simulink model "BEV_maxSpeed"  (R2023a)
settings: Solver=FixedStepAuto  StartTime=0.0  StopTime=1000  FixedStep=1  RelTol=1e-3
undefined symbols (not defined in the file): acceleration_threshold, attributes, battery_GD, config_gearbox, config_Inverter, config_motor, config_vehicle, efficiency_vector, efficiency_vector2, GB, gearbox_map, k_FW, lossData, lossData2, max_torque_map, max_torque_map2, speed_vector, speed_vector2
libraries: spsParallelRLCBranchLib x20, spsControlledCurrentSourceLib x8, spsVoltageMeasurementLib x8, simulink x4, spsDCVoltageSourceLib x4, spspowerguiLib x4, eePmsmCurrentReferenceGen x2
(part 2 of 2)

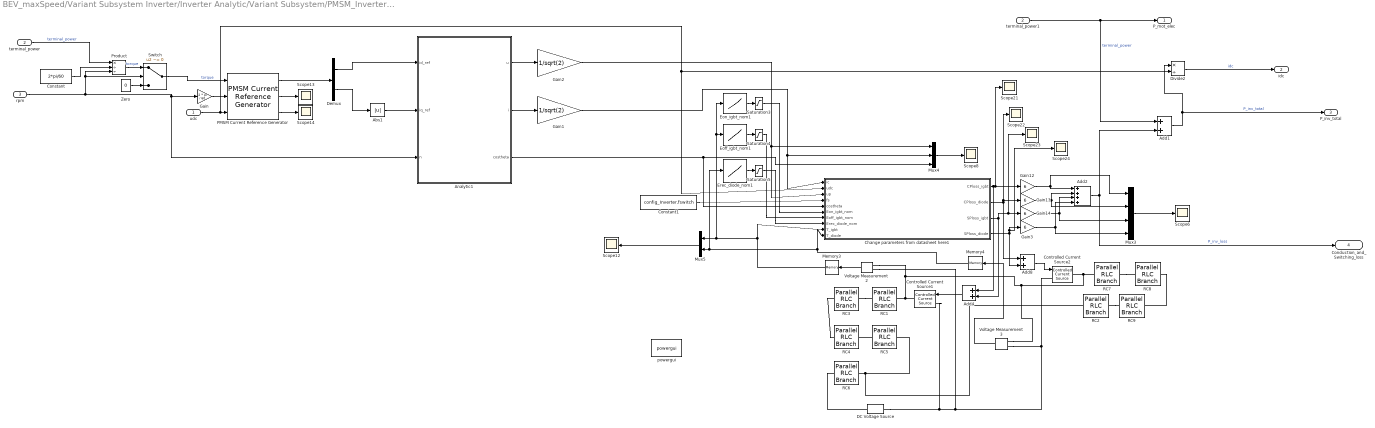
== system BEV_maxSpeed/Variant Subsystem Inverter/Inverter Analytic/Variant Subsystem/PMSM_Inverter_IBGT_Analytic ==
  udc : Inport
  terminal_power : Inport  Port=2
  rpm : Inport  Port=3
  Abs1 : Abs  SaturateOnIntegerOverflow=off
  Add1 : Sum
  Add2 : Sum  Inputs=++++
  Add4 : Sum
  Add8 : Sum
  Analytic1 : MATLAB Function  TreatAsAtomicUnit=on
  Change parameters from datasheet here1 : MATLAB Function  TreatAsAtomicUnit=on
  Constant : Constant  Value=2*pi/60
  Constant1 : Constant  Value=config_Inverter.fswitch
  Controlled Current Source1 : spsControlledCurrentSourceLib/Controlled Current Source  Initialize=on  Source_Type=AC  Amplitude=0  Phase=0  Frequency=0  Measurements=None
  Controlled Current Source2 : spsControlledCurrentSourceLib/Controlled Current Source  Initialize=on  Source_Type=AC  Amplitude=0  Phase=0  Frequency=0  Measurements=None
  DC Voltage Source : spsDCVoltageSourceLib/DC Voltage Source  Amplitude=25  Measurements=None
  Demux : Demux  Outputs=2
  Divide2 : Product  Inputs=*/
  Eoff_igbt_nom1 : Lookup_n-D  NumberOfTableDimensions=1  BreakpointsForDimension1=[25, 150, 175]  Table="[23.5*1e-3,  29*1e-3,  30*1e-3]"  InternalRulePriority=Speed  RndMeth=Simplest
  Eon_igbt_nom1 : Lookup_n-D  NumberOfTableDimensions=1  BreakpointsForDimension1=[25, 150, 175]  Table="[13.5*1e-3,  17.5*1e-3,  18*1e-3]"  InternalRulePriority=Speed  RndMeth=Simplest
  Erec_diode_nom1 : Lookup_n-D  NumberOfTableDimensions=1  BreakpointsForDimension1=[25, 150, 175]  Table="[7*1e-3,  13*1e-3,  15*1e-3]"  InternalRulePriority=Speed  RndMeth=Simplest
  Gain : Gain  Gain=2 * pi / 60
  Gain1 : Gain  Gain=1/sqrt(2)
  Gain{3,12..14} (4 alike) : Gain  Gain=6
  Gain2 : Gain  Gain=1/sqrt(2)
  Memory3 : Memory  InitialCondition=25  InheritSampleTime=on
  Memory4 : Memory  InitialCondition=25  InheritSampleTime=on
  Mux3 : Mux
  Mux4 : Mux  Inputs=3
  Mux5 : Mux  Inputs=2
  PMSM Current Reference Generator : eePmsmCurrentReferenceGen/PMSM Current Reference Generator  Vnom=360  Pmax=150000  Tmax=350  Ts=-1  RefType=Automatically generated lookup-table  rpmVec=[0, 3000]  TqVec=[-100, 0, 100]  VdcVec=[300, 350]  PWMMode=SPWM: sinusoidal PWM  ModFactor=0.97  idMatrix=zeros(2,3,2)  iqMatrix=zeros(2,3,2)  p=6  psim=0.0347  Ld=0.0000436  Lq=0.0000975  Rs=0.0049  RefExpEnable=0
      settings: LibrarySourceBlock=|
      | ee_sl_lib/PMSM Control/PMSM Current Reference
      | Generator
  Product : Product  Inputs=*//
  RC1 : spsParallelRLCBranchLib/Parallel RLC Branch  LConnTagsString=a  RConnTagsString=__new0  BranchType=RC  Resistance=config_Inverter.R1igbt  Inductance=1e-3  SetiL0=off  InitialCurrent=0  Capacitance=config_Inverter.C1igbt  Setx0=off  InitialVoltage=0  Measurements=None
  RC2 : spsParallelRLCBranchLib/Parallel RLC Branch  LConnTagsString=a  RConnTagsString=__new0  BranchType=RC  Resistance=config_Inverter.R4diode  Inductance=1e-3  SetiL0=off  InitialCurrent=0  Capacitance=config_Inverter.C4diode  Setx0=off  InitialVoltage=0  Measurements=None
  RC3 : spsParallelRLCBranchLib/Parallel RLC Branch  LConnTagsString=a  RConnTagsString=__new0  BranchType=RC  Resistance=config_Inverter.R2igbt  Inductance=1e-3  SetiL0=off  InitialCurrent=0  Capacitance=config_Inverter.C2igbt  Setx0=off  InitialVoltage=0  Measurements=None
  RC4 : spsParallelRLCBranchLib/Parallel RLC Branch  LConnTagsString=a  RConnTagsString=__new0  BranchType=RC  Resistance=config_Inverter.R3igbt  Inductance=1e-3  SetiL0=off  InitialCurrent=0  Capacitance=config_Inverter.C3igbt  Setx0=off  InitialVoltage=0  Measurements=None
  RC5 : spsParallelRLCBranchLib/Parallel RLC Branch  LConnTagsString=a  RConnTagsString=__new0  BranchType=RC  Resistance=config_Inverter.R4igbt  Inductance=1e-3  SetiL0=off  InitialCurrent=0  Capacitance=config_Inverter.C4igbt  Setx0=off  InitialVoltage=0  Measurements=None
  RC6 : spsParallelRLCBranchLib/Parallel RLC Branch  LConnTagsString=a  RConnTagsString=__new0  BranchType=R  Resistance=config_Inverter.R6igbt  Inductance=1e-3  SetiL0=off  InitialCurrent=0  Capacitance=175  Setx0=on  InitialVoltage=0  Measurements=None
  RC7 : spsParallelRLCBranchLib/Parallel RLC Branch  LConnTagsString=a  RConnTagsString=__new0  BranchType=RC  Resistance=config_Inverter.R1diode  Inductance=1e-3  SetiL0=off  InitialCurrent=0  Capacitance=config_Inverter.C1diode  Setx0=off  InitialVoltage=0  Measurements=None
  RC8 : spsParallelRLCBranchLib/Parallel RLC Branch  LConnTagsString=a  RConnTagsString=__new0  BranchType=RC  Resistance=config_Inverter.R2diode  Inductance=1e-3  SetiL0=off  InitialCurrent=0  Capacitance=config_Inverter.C2diode  Setx0=off  InitialVoltage=0  Measurements=None
  RC9 : spsParallelRLCBranchLib/Parallel RLC Branch  LConnTagsString=a  RConnTagsString=__new0  BranchType=RC  Resistance=config_Inverter.R3diode  Inductance=1e-3  SetiL0=off  InitialCurrent=0  Capacitance=config_Inverter.C3diode  Setx0=off  InitialVoltage=0  Measurements=None
  Saturation3 : Saturate  UpperLimit=18*1e-3  LowerLimit=13.5*1e-3
  Saturation4 : Saturate  UpperLimit=30*1e-3  LowerLimit=23.5*1e-3
  Saturation5 : Saturate  UpperLimit=15*1e-3  LowerLimit=7*1e-3
  Scope{6,8,12..14,21..24} (9 alike) : Scope
  Switch : Switch  Criteria=u2 ~= 0  SaturateOnIntegerOverflow=off  InputSameDT=off
  Voltage Measurement2 : spsVoltageMeasurementLib/Voltage Measurement  PhasorSimulation=off  OutputType=Complex  PSBequivalent=0
  Voltage Measurement3 : spsVoltageMeasurementLib/Voltage Measurement  PhasorSimulation=off  OutputType=Complex  PSBequivalent=0
  Zero : Constant  Value=0  OutDataTypeStr=Inherit: Inherit via back propagation
  powergui : spspowerguiLib/powergui  Priority=1  SimulationMode=Discrete  SampleTime=1  frequency=60  Iterations=50  frequencyindice=0  Pbase=100e6  ErrMax=1e-4  UnitsV=kV  UnitsW=MW  buscounter=0  FunctionMessages=on  echomessages=on  EnableUseOfTLC=off  CurrentSourceSwitches=off  DisableSnubberDevices=off  DisableRonSwitches=off  DisableVfSwitches=off  DisplayEquations=off  AutomaticDiscreteSolvers=off  SolverType=Backward Euler  Interpol=off  ExternalGateDelay=off  methode=off  Ts=100  x0status=blocks  SPID=off  SwTol=0  HookPort=off  NonlinearTolerance=1e-4  nMaxIteration=100  ContinueOnMaxIteration=off  RestoreLinks=warning  ResistiveCurrentMeasurement=off  Frange=[0:2:500]  Ylog=off  Xlog=on  ShowGrid=off  save=off  variable=ZData  structure=0  ZoomFFT=off  StartTime=0.0  cycles=1  DisplayStyle=1  fundamental=60  FreqAxis=off  MaxFrequency=1000  frequencyindicesteady=1  RmsSteady=1  display=off
  terminal_power1 : InportShadow  Port=2
  P_mot_elec : Outport
  idc : Outport  Port=2
  P_inv_total : Outport  Port=3
  Conduction_and_Switching_loss : Outport  Port=4
  wires:
  PMSM Current Reference Generator/2 -> Scope13/1
  Eon_igbt_nom1/1 -> Saturation3/1
  Divide2/1 -> idc/1  "idc"
  Voltage Measurement2/1 -> Memory3/1
  Add8/1 -> Controlled Current Source2/1
  Change parameters from datasheet here1/3(SPloss_igbt) -> Scope23/1, Gain14/1, Add4/2
  Change parameters from datasheet here1/1(CPloss_igbt) -> Add4/1, Gain12/1, Scope21/1
  Gain2/1 -> Change parameters from datasheet here1/3(up), Mux4/1
  Add4/1 -> Controlled Current Source1/1
  Constant1/1 -> Change parameters from datasheet here1/4(fs)
  Eoff_igbt_nom1/1 -> Saturation4/1
  Saturation4/1 -> Change parameters from datasheet here1/7(Eoff_igbt_nom)
  PMSM Current Reference Generator/3 -> Scope14/1
  Demux/2 -> Abs1/1
  Change parameters from datasheet here1/2(CPloss_diode) -> Scope22/1, Gain13/1, Add8/1
  Voltage Measurement3/1 -> Memory4/1
  Memory3/1 -> Change parameters from datasheet here1/9(T_igbt), Eoff_igbt_nom1/1, Eon_igbt_nom1/1, Mux5/1
  Mux4/1 -> Scope8/1
  Mux5/1 -> Scope12/1
  Demux/1 -> Analytic1/1(id_ref)
  Memory4/1 -> Erec_diode_nom1/1, Mux5/2, Change parameters from datasheet here1/10(T_diode)
  Saturation5/1 -> Change parameters from datasheet here1/8(Erec_diode_nom)
  Add1/1 -> Divide2/1, P_inv_total/1  "P_inv_total"
  Analytic1/1(u) -> Gain2/1
  Erec_diode_nom1/1 -> Saturation5/1
  Mux3/1 -> Scope6/1
  Gain14/1 -> Mux3/3, Add2/3
  Gain/1 -> PMSM Current Reference Generator/2
  Add2/1 -> Conduction_and_Switching_loss/1, Add1/2  "P_inv_loss"
  Change parameters from datasheet here1/4(SPloss_diode) -> Scope24/1, Gain3/1, Add8/2
  Analytic1/2(i) -> Gain1/1
  PMSM Current Reference Generator/1 -> Demux/1
  Saturation3/1 -> Change parameters from datasheet here1/6(Eon_igbt_nom)
  Abs1/1 -> Analytic1/2(iq_ref)
  Gain13/1 -> Mux3/2, Add2/2
  rpm/1 -> Switch/2, Product/3, Analytic1/3(n), Gain/1
  terminal_power1/1 -> P_mot_elec/1, Add1/1  "terminal_power"
  Gain1/1 -> Change parameters from datasheet here1/1(ic), Mux4/2
  Gain12/1 -> Mux3/1, Add2/1
  udc/1 -> PMSM Current Reference Generator/3, Change parameters from datasheet here1/2(udc), Divide2/2
  Switch/1 -> PMSM Current Reference Generator/1  "torque"
  Gain3/1 -> Add2/4, Mux3/4
  Analytic1/3(costheta) -> Mux4/3, Change parameters from datasheet here1/5(costheta)
  terminal_power/1 -> Product/1  "terminal_power"
  Constant/1 -> Product/2
  Product/1 -> Switch/1  "torque"
  Zero/1 -> Switch/3
  connections:
  RC3/RConn1 -- RC1/LConn1
  RC7/LConn1 -- RC8/RConn1
  DC Voltage Source/RConn1 -- RC6/LConn1
  RC3/LConn1 -- RC4/LConn1
  RC5/LConn1 -- RC4/RConn1
  RC8/LConn1 -- RC9/LConn1
  Controlled Current Source1/LConn1 -- DC Voltage Source/LConn1 -- Voltage Measurement2/LConn1 -- Voltage Measurement3/LConn1 -- Controlled Current Source2/LConn1
  RC2/LConn1 -- RC9/RConn1
  RC5/RConn1 -- RC6/RConn1 -- RC2/RConn1
  Controlled Current Source2/RConn1 -- RC7/RConn1 -- Voltage Measurement3/LConn2 -- Voltage Measurement2/LConn2 -- Controlled Current Source1/RConn1 -- RC1/RConn1

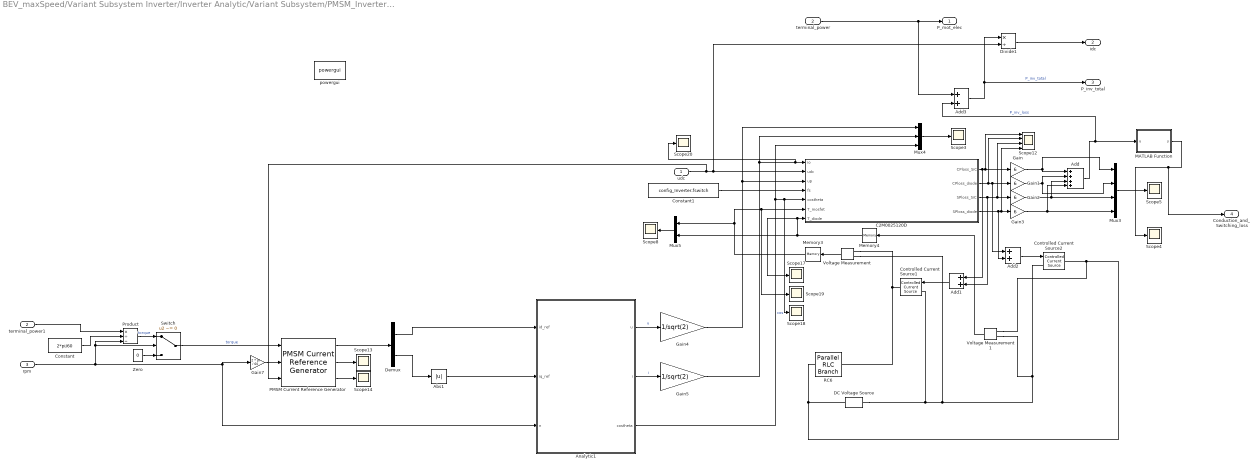
== system BEV_maxSpeed/Variant Subsystem Inverter/Inverter Analytic/Variant Subsystem/PMSM_Inverter_SiC-MOSFET_Analytic ==
  udc : Inport
  terminal_power : Inport  Port=2
  rpm : Inport  Port=3
  Abs1 : Abs  SaturateOnIntegerOverflow=off
  Add : Sum  Inputs=++++
  Add1 : Sum
  Add2 : Sum
  Add3 : Sum
  Analytic1 : MATLAB Function  TreatAsAtomicUnit=on
  C2M0025120D : MATLAB Function  TreatAsAtomicUnit=on
  Constant : Constant  Value=2*pi/60
  Constant1 : Constant  Value=config_Inverter.fswitch
  Controlled Current Source1 : spsControlledCurrentSourceLib/Controlled Current Source  Initialize=on  Source_Type=AC  Amplitude=0  Phase=0  Frequency=0  Measurements=None
  Controlled Current Source2 : spsControlledCurrentSourceLib/Controlled Current Source  Initialize=on  Source_Type=AC  Amplitude=0  Phase=0  Frequency=0  Measurements=None
  DC Voltage Source : spsDCVoltageSourceLib/DC Voltage Source  Amplitude=25  Measurements=None
  Demux : Demux  Outputs=2
  Divide1 : Product  Inputs=*/
  Gain{,1..3} (4 alike) : Gain  Gain=6
  Gain4 : Gain  Gain=1/sqrt(2)
  Gain5 : Gain  Gain=1/sqrt(2)
  Gain7 : Gain  Gain=2 * pi / 60
  MATLAB Function : MATLAB Function  TreatAsAtomicUnit=on
  Memory3 : Memory  InitialCondition=25  InheritSampleTime=on
  Memory4 : Memory  InitialCondition=25  InheritSampleTime=on
  Mux3 : Mux
  Mux4 : Mux  Inputs=3
  Mux5 : Mux  Inputs=2
  PMSM Current Reference Generator : eePmsmCurrentReferenceGen/PMSM Current Reference Generator  Vnom=360  Pmax=150000  Tmax=350  Ts=-1  RefType=Automatically generated lookup-table  rpmVec=[0, 3000]  TqVec=[-100, 0, 100]  VdcVec=[300, 350]  PWMMode=SPWM: sinusoidal PWM  ModFactor=0.97  idMatrix=zeros(2,3,2)  iqMatrix=zeros(2,3,2)  p=6  psim=0.0347  Ld=0.0000436  Lq=0.0000975  Rs=0.0049  RefExpEnable=0
      settings: LibrarySourceBlock=|
      | ee_sl_lib/PMSM Control/PMSM Current Reference
      | Generator
  Product : Product  Inputs=*//
  RC6 : spsParallelRLCBranchLib/Parallel RLC Branch  LConnTagsString=a  RConnTagsString=__new0  BranchType=R  Resistance=config_Inverter.Rmosfet  Inductance=1e-3  SetiL0=off  InitialCurrent=0  Capacitance=175  Setx0=on  InitialVoltage=0  Measurements=None
  Scope12 : Scope  NumInputPorts=4
  Scope{3..5,8,13..14,17..20} (10 alike) : Scope
  Switch : Switch  Criteria=u2 ~= 0  SaturateOnIntegerOverflow=off  InputSameDT=off
  Voltage Measurement : spsVoltageMeasurementLib/Voltage Measurement  PhasorSimulation=off  OutputType=Complex  PSBequivalent=0
  Voltage Measurement1 : spsVoltageMeasurementLib/Voltage Measurement  PhasorSimulation=off  OutputType=Complex  PSBequivalent=0
  Zero : Constant  Value=0  OutDataTypeStr=Inherit: Inherit via back propagation
  powergui : spspowerguiLib/powergui  Priority=1  SimulationMode=Discrete  SampleTime=1  frequency=60  Iterations=50  frequencyindice=0  Pbase=100e6  ErrMax=1e-4  UnitsV=kV  UnitsW=MW  buscounter=0  FunctionMessages=on  echomessages=on  EnableUseOfTLC=off  CurrentSourceSwitches=off  DisableSnubberDevices=off  DisableRonSwitches=off  DisableVfSwitches=off  DisplayEquations=off  AutomaticDiscreteSolvers=off  SolverType=Backward Euler  Interpol=off  ExternalGateDelay=off  methode=off  Ts=100  x0status=blocks  SPID=off  SwTol=0  HookPort=off  NonlinearTolerance=1e-4  nMaxIteration=100  ContinueOnMaxIteration=off  RestoreLinks=warning  ResistiveCurrentMeasurement=off  Frange=[0:2:500]  Ylog=off  Xlog=on  ShowGrid=off  save=off  variable=ZData  structure=0  ZoomFFT=off  StartTime=0.0  cycles=1  DisplayStyle=1  fundamental=60  FreqAxis=off  MaxFrequency=1000  frequencyindicesteady=1  RmsSteady=1  display=off
  terminal_power1 : InportShadow  Port=2
  P_mot_elec : Outport
  idc : Outport  Port=2
  P_inv_total : Outport  Port=3
  Conduction_and_Switching_loss : Outport  Port=4
  wires:
  udc/1 -> PMSM Current Reference Generator/3, Divide1/2, C2M0025120D/2(udc)
  Gain1/1 -> Mux3/2, Add/2
  Gain4/1 -> Mux4/1, C2M0025120D/3(up)
  Memory3/1 -> Mux5/1, Scope19/1, C2M0025120D/6(T_mosfet)
  Add2/1 -> Controlled Current Source2/1
  Constant1/1 -> C2M0025120D/4(fs)
  Divide1/1 -> idc/1
  C2M0025120D/3(SPloss_SiC) -> Add1/2, Scope12/3, Gain2/1
  Analytic1/3(costheta) -> Mux4/3, Scope18/1, C2M0025120D/5(costheta)  "cos"
  Gain/1 -> Mux3/1, Add/1
  C2M0025120D/2(CPloss_diode) -> Scope12/2, Add2/1, Gain1/1
  Mux4/1 -> Scope3/1
  Gain5/1 -> Mux4/2, Scope20/1, C2M0025120D/1(io)
  terminal_power/1 -> P_mot_elec/1, Add3/1
  Memory4/1 -> Scope17/1, C2M0025120D/7(T_diode), Mux5/2
  Add/1 -> Add3/2, MATLAB Function/1(u)  "P_inv_loss"
  C2M0025120D/4(SPloss_diode) -> Scope12/4, Gain3/1, Add2/2
  Gain2/1 -> Mux3/3, Add/3
  Add1/1 -> Controlled Current Source1/1
  C2M0025120D/1(CPloss_SiC) -> Add1/1, Scope12/1, Gain/1
  Analytic1/2(i) -> Gain5/1  "i"
  Gain3/1 -> Add/4, Mux3/4
  Voltage Measurement1/1 -> Memory4/1
  Add3/1 -> P_inv_total/1, Divide1/1  "P_inv_total"
  Voltage Measurement/1 -> Memory3/1
  Mux5/1 -> Scope8/1
  Mux3/1 -> Scope5/1
  Analytic1/1(u) -> Gain4/1  "u"
  PMSM Current Reference Generator/3 -> Scope14/1
  PMSM Current Reference Generator/2 -> Scope13/1
  Switch/1 -> PMSM Current Reference Generator/1  "torque"
  Demux/2 -> Abs1/1
  rpm/1 -> Gain7/1, Analytic1/3(n), Switch/2, Product/3
  Gain7/1 -> PMSM Current Reference Generator/2
  Demux/1 -> Analytic1/1(id_ref)
  Abs1/1 -> Analytic1/2(iq_ref)
  PMSM Current Reference Generator/1 -> Demux/1
  Zero/1 -> Switch/3
  Constant/1 -> Product/2
  Product/1 -> Switch/1  "torque"
  terminal_power1/1 -> Product/1
  MATLAB Function/1(y) -> Conduction_and_Switching_loss/1, Scope4/1
  connections:
  Voltage Measurement/LConn1 -- Controlled Current Source1/RConn1 -- RC6/RConn1
  DC Voltage Source/RConn1 -- Controlled Current Source2/RConn1 -- Voltage Measurement1/LConn1 -- RC6/LConn1
  Voltage Measurement1/LConn2 -- DC Voltage Source/LConn1 -- Controlled Current Source1/LConn1 -- Voltage Measurement/LConn2 -- Controlled Current Source2/LConn1

== system BEV_maxSpeed/Variant Subsystem Gearbox/Gearbox Analytic/Variant Subsystem Analytic GB/Einstufig_Achsparallel/Ölpumpe ==
  nrad : Inport
  Constant : Constant  Value=config_gearbox.power_oilpump
  Constant1 : Constant  Value=1.5e3
  Product : Product  Inputs=*/*
  Scope : Scope
  power_oilpump : Outport
  wires:
  Product/1 -> power_oilpump/1, Scope/1
  Constant1/1 -> Product/2
  nrad/1 -> Product/1
  Constant/1 -> Product/3

== system BEV_maxSpeed/Variant Subsystem Gearbox/Gearbox Analytic/Variant Subsystem Analytic GB/Zweistufig_Achsparallel/Ölpumpe ==
  nrad : Inport
  Constant : Constant  Value=config_gearbox.power_oilpump
  Constant1 : Constant  Value=15e3
  Product : Product  Inputs=*/*
  Scope : Scope
  power_oilpump : Outport
  wires:
  Product/1 -> power_oilpump/1, Scope/1
  Constant1/1 -> Product/2
  nrad/1 -> Product/1
  Constant/1 -> Product/3

== system BEV_maxSpeed/Variant Subsystem Gearbox/Gearbox Analytic/Variant Subsystem Analytic GB/Zweistufig_Koaxial/Ölpumpe ==
  nrad : Inport
  Constant : Constant  Value=config_gearbox.power_oilpump
  Constant1 : Constant  Value=1.5e3
  Product : Product  Inputs=*/*
  Scope : Scope
  power_oilpump : Outport
  wires:
  Product/1 -> power_oilpump/1, Scope/1
  Constant1/1 -> Product/2
  nrad/1 -> Product/1
  Constant/1 -> Product/3

== system BEV_maxSpeed/Variant Subsystem Gearbox/Gearbox Lookup-Table/Variant Subsystem/ETA_map/Lookup Gearbox ==
  note: 1) Add Subsystem or Model blocks as valid variant choices.
      | 2) You cannot connect blocks at this level. At simulation, connectivity is automatically
      | determined, based on the active variant and port name matching.
  Torque : Inport
  RPM : Inport  Port=2
  Temp : Inport  Port=3
  Lookup with Temp : Subsystem  VariantControl=gearbox_map.dim_lookup == 3
  Lookup without Temp : Subsystem  VariantControl=gearbox_map.dim_lookup == 2
  Eta : Outport

== system BEV_maxSpeed/Variant Subsystem Gearbox/Gearbox Lookup-Table/Variant Subsystem/ETA_map/Oilpump ==
  rpm_wheel : Inport
  Constant7 : Constant  Value=config_gearbox.power_oilpump
  Constant8 : Constant  Value=1.5e3
  Product4 : Product  Inputs=**/
  loss_oilpump : Outport
  wires:
  rpm_wheel/1 -> Product4/1
  Constant8/1 -> Product4/3
  Constant7/1 -> Product4/2
  Product4/1 -> loss_oilpump/1  "loss_oilpump"

== system BEV_maxSpeed/Variant Subsystem Gearbox/Gearbox Lookup-Table/Variant Subsystem/LOSS_map/Lookup Gearbox ==
  note: 1) Add Subsystem or Model blocks as valid variant choices.
      | 2) You cannot connect blocks at this level. At simulation, connectivity is automatically
      | determined, based on the active variant and port name matching.
  Torque : Inport
  RPM : Inport  Port=2
  Temp : Inport  Port=3
  Lookup with Temp : Subsystem  VariantControl=gearbox_map.dim_lookup == 3
  Lookup without Temp : Subsystem  VariantControl=gearbox_map.dim_lookup == 2
  Loss : Outport

== system BEV_maxSpeed/Variant Subsystem Gearbox/Gearbox Lookup-Table/Variant Subsystem/LOSS_map/Oilpump ==
  rpm_wheel : Inport
  Constant7 : Constant  Value=config_gearbox.power_oilpump
  Constant8 : Constant  Value=1.5e3
  Product4 : Product  Inputs=**/
  loss_oilpump : Outport
  wires:
  Product4/1 -> loss_oilpump/1  "loss_oilpump"
  Constant7/1 -> Product4/2
  Constant8/1 -> Product4/3
  rpm_wheel/1 -> Product4/1

== system BEV_maxSpeed/Variant Subsystem Gearbox/Gearbox Lookup-Table/Variant Subsystem/ETA_map/Lookup Gearbox/Lookup with Temp ==
  Torque : Inport
  RPM : Inport  Port=2
  Temp : Inport  Port=3
  n-D Lookup Table : Lookup_n-D  NumberOfTableDimensions=3  BreakpointsForDimension1=gearbox_map.torque  BreakpointsForDimension2=gearbox_map.rpm  BreakpointsForDimension3=gearbox_map.temperature  Table=gearbox_map.eta  UseLastTableValue=on  InternalRulePriority=Speed  RndMeth=Simplest
      settings: InputPortMap=u0,u1,u2
  Eta : Outport
  wires:
  Torque/1 -> n-D Lookup Table/1
  RPM/1 -> n-D Lookup Table/2
  Temp/1 -> n-D Lookup Table/3
  n-D Lookup Table/1 -> Eta/1

== system BEV_maxSpeed/Variant Subsystem Gearbox/Gearbox Lookup-Table/Variant Subsystem/ETA_map/Lookup Gearbox/Lookup without Temp ==
  Torque : Inport
  RPM : Inport  Port=2
  n-D Lookup Table : Lookup_n-D  BreakpointsForDimension1=gearbox_map.torque  BreakpointsForDimension2=gearbox_map.rpm  BreakpointsForDimension3=gearbox_map.temperature  Table=gearbox_map.eta  UseLastTableValue=on  InternalRulePriority=Speed  RndMeth=Simplest
      settings: InputPortMap=u0,u1
  Eta : Outport
  wires:
  Torque/1 -> n-D Lookup Table/1
  RPM/1 -> n-D Lookup Table/2
  n-D Lookup Table/1 -> Eta/1

== system BEV_maxSpeed/Variant Subsystem Gearbox/Gearbox Lookup-Table/Variant Subsystem/LOSS_map/Lookup Gearbox/Lookup with Temp ==
  Torque : Inport
  RPM : Inport  Port=2
  Temp : Inport  Port=3
  n-D Lookup Table : Lookup_n-D  NumberOfTableDimensions=3  BreakpointsForDimension1=gearbox_map.torque  BreakpointsForDimension2=gearbox_map.rpm  BreakpointsForDimension3=gearbox_map.temperature  Table=gearbox_map.loss  UseLastTableValue=on  InternalRulePriority=Speed  RndMeth=Simplest
      settings: InputPortMap=u0,u1,u2
  Loss : Outport
  wires:
  n-D Lookup Table/1 -> Loss/1
  Temp/1 -> n-D Lookup Table/3
  RPM/1 -> n-D Lookup Table/2
  Torque/1 -> n-D Lookup Table/1

== system BEV_maxSpeed/Variant Subsystem Gearbox/Gearbox Lookup-Table/Variant Subsystem/LOSS_map/Lookup Gearbox/Lookup without Temp ==
  Torque : Inport
  RPM : Inport  Port=2
  n-D Lookup Table : Lookup_n-D  BreakpointsForDimension1=gearbox_map.torque  BreakpointsForDimension2=gearbox_map.rpm  BreakpointsForDimension3=gearbox_map.temperature  Table=gearbox_map.loss  UseLastTableValue=on  InternalRulePriority=Speed  RndMeth=Simplest
      settings: InputPortMap=u0,u1
  Loss : Outport
  wires:
  n-D Lookup Table/1 -> Loss/1
  RPM/1 -> n-D Lookup Table/2
  Torque/1 -> n-D Lookup Table/1

== matlab function BEV_maxSpeed/MATLAB Function ==
  data: availble_torque_acc_motor input; a output; iges input; tire_radius input; mass_total input
function a = fcn(availble_torque_acc_motor, iges, tire_radius, mass_total)

 torque_wheel = availble_torque_acc_motor * iges;

 F_net = torque_wheel / tire_radius;

 a = F_net / mass_total;

== matlab function BEV_maxSpeed/MATLAB Function1 ==
  data: a input; dt input; v_new output; v_prev input; time_prev input; time_new output
function [v_new, time_new] = update_velocity(a, dt, v_prev, time_prev)
    % Inputs:
    % a          - Acceleration (input signal)
    % dt         - Time step (constant or input signal)
    % v_prev     - Previous velocity (feedback input)
    % time_prev  - Previous time (feedback input)

    % Outputs:
    % v_new     - Updated velocity
    % time_new  - Updated time

    % Calculate new velocity using v = u + a * dt
    v_new = v_prev + a * dt;

    % Update time
    time_new = time_prev + dt;
end

== matlab function BEV_maxSpeed/Variant Subsystem Inverter/Inverter Analytic/Variant Subsystem/IM_Inverter_IGBT_Analytic/MATLAB Function3 ==
  data: u output; T_m input; i output; usq input; usd input; costheta output; n input
function [u, i, costheta] = fcn(T_m, usq, usd, n)

   Lm = 4.5e-4;
   Lr =  0.01571 + Lm;
   p = 3;
   T_e = T_m/p;
   
   if T_m >=0
       id = -sqrt((2*T_e/p*Lr)/(3*p*Lm^2));
   else
       id = sqrt((-2*T_e/p*Lr)/(3*p*Lm^2));
   end
   iq = id;
   i = sqrt(id^2 + iq^2)/2;
   u = sqrt(usq*usq+usd*usd);
   costheta = (usd*id+usq*iq)/u/i;

   if isnan(costheta)
       costheta = 1;
   end

   if n < 0.1
       u = 0;
       i = 0;
       costheta = 1;
   end

end

== matlab function BEV_maxSpeed/Variant Subsystem Inverter/Inverter Analytic/Variant Subsystem/IM_Inverter_SiC-MOSFET_Analytic/MATLAB Function ==
  data: t input; udc input; w_mech input; u_sq output; u_sd output
function [u_sq, u_sd] = fcn(t, udc, w_mech)
    
    p = 3; %pole pairs
    
    V_line = udc/2;
    V_phase = V_line/sqrt(3);
    w_elect = p * w_mech;
    
    V_a = V_phase * sin(w_elect * t);
    V_b = V_phase * sin(w_elect * t - 2*pi/3);
    V_c = V_phase * sin(w_elect * t + 2*pi/3);

    % Transformation from abc to dq reference frame
    % Assuming stator flux-oriented control with d-axis aligned with rotor flux
    theta_e = w_elect * t; % Electrical angle
    
    % Clarke transformation to alpha-beta reference frame
    V_alpha = (2/3) * (V_a - 0.5 * (V_b + V_c));
    V_beta = (2/3) * ((sqrt(3)/2) * (V_b - V_c));
    
    % Park transformation to d-q reference frame
    u_sd = V_alpha * cos(theta_e) + V_beta * sin(theta_e);
    u_sq = -V_alpha * sin(theta_e) + V_beta * cos(theta_e);

end

== matlab function BEV_maxSpeed/Variant Subsystem Gearbox/Gearbox Lookup-Table/Oil Temp/MATLAB Function ==
  data: t input; P_V input; T output
function T = fcn(t, P_V)

coder.extrinsic('evalin');

% Calculate lubricant temperature
ambient_temp = 0;
ambient_temp = evalin('base', 'config_vehicle.ambient_temp');
% 
% if t < (ambient_temp - 273)
%     T = (ambient_temp - 273);
% elseif t <= 70 %Aufwärmphase mit Umgebung < t < 70°C
%     T = abs(P) * 0.0003 + rpm * 0.00004 + t; %Leistungsabhängiger und drehzahlabhängiger Energieeintrag (Temperaturanstieg)
% else %Temperatur t > 70°C -> Wärmeabgabe ~ delta_t und ~ delta_t^2 (mit delta_t = t_gearbox - t_ambient)
%     T = abs(P) * 0.0003 + rpm * 0.00004 + t - (t - ambient_temp + 273) * 0.0002 - (t - ambient_temp + 273)^2 * 0.0000022;
% end

if t < (ambient_temp - 273)
    T = (ambient_temp - 273);
elseif t <= 80 %Aufwärmphase mit Umgebung < t < 70°C
    T =0.000055*P_V + t - (t - ambient_temp + 273) * 0.0003; %Leistungsabhängiger und drehzahlabhängiger Energieeintrag (Temperaturanstieg)
else %Temperatur t > 70°C -> Wärmeabgabe ~ delta_t und ~ delta_t^2 (mit delta_t = t_gearbox - t_ambient)
    T = 0.000088*P_V + t - (t - ambient_temp + 273) * 0.0010 - (t - ambient_temp + 273)^2 * 0.000012;
end

end

== matlab function BEV_maxSpeed/Variant Subsystem Inverter/Inverter Analytic/Variant Subsystem/PMSM_Inverter_SiC-MOSFET_Analytic/MATLAB Function ==
  data: u input; y output
function y = fcn(u)
    if isnan(u)
        warning('P_inveter_loss is NaN. ');
  
    end

    y=u;

== matlab function BEV_maxSpeed/Variant Subsystem Inverter/Inverter Analytic/Variant Subsystem/IM_Inverter_SiC-MOSFET_Analytic/C2M0025120D ==
  data: io input; udc input; up input; fs input; CPloss_SiC output; CPloss_diode output; costheta input; SPloss_SiC output; SPloss_diode output; T_mosfet input; T_diode input
function [CPloss_SiC,CPloss_diode,SPloss_SiC,SPloss_diode] = SiC_MOSFET(io,udc,up,fs,costheta,T_mosfet,T_diode)
%%%%%%%%%%%%%%%%%%%%%%%%%%% parameter table %%%%%%%%%%%%%%%%%%%%%%%%%%%%%%%
%%%%%%%%%%%%%%%%%%%%%%%%%%% varialbe table %%%%%%%%%%%%%%%%%%%%%%%%%%%%%%%%
%variavle name      meaning,                                                        unit
%io,                operation current                                               (A)
%up,                operation voltage                                               (V)
%udc,               DC bus voltage,                                                 (V)
%fs,                switching frequency,                                            (Hz)
%costheta,          power factor,                                                   (none)
%CPloss_igbt,       conduction loss on IGBT,                                        (W)
%CPloss_diode,      conduction loss on the reverse paralleled diode,                (W)
%SPloss_igbt,       switching loss on IGBT,                                         (W)
%SPloss_diode,      switching loss on the reverse paralleled diode,                 (W)
%%%%%%%%%%%%%%%%%%%%%%%%%%%%%%%%%%%%%%%%%%%%%%%%%%%%%%%%%%%%%%%%%%%%%%%%%%%
parallel = 4;

io = io/parallel;
rdson_max = 0.02;       
alpha = (1.45 - 1)/(150 - 25);
ud_plateau25 = 1;                              % Fig.11; Vth,25 = 2.7
ud_plateau150 = 0.717;                         % Fig.11; Vth,150 = 2.3
%%%%%%%%%%%%%%%%%%%%%%%%%%%% linearization %%%%%%%%%%%%%%%%%%%%%%%%%%%%%%%%
rdson = rdson_max*(1 + alpha/100)^(T_mosfet - 25);
ud_plateau = ud_plateau25 + (ud_plateau25-ud_plateau150)/(25-150)*(T_diode-25);

rd = (-6 - (-3.75))/(-200 - 0) * 1.2;          % engineering calculation use safty margin value, linearization from Fig.10, using Vsd,typ = 3.5;

Eon_SiC = (0.00069/80*(io*(2/pi)))/520*udc;    % linearization from Fig.23; V_DD = 600; Eon(60, 0.0015);
Eoff_SiC = (0.001125/80*(io*(2/pi)))/520*udc;  % linearization from Fig.23; V_DD = 600; Eoff(60, 0.00075);
Eon_diode = 0;
Eoff_diode = 0;
%%%%%%%%%%%%%%%%%%%%%%%%%%%%%%%%%%%%%%%%%%%%%%%%%%%%%%%%%%%%%%%%%%%%%%%%%%%
m = sqrt(2)*up*2/udc;

if io*rdson <= ud_plateau
   CPloss_SiC = rdson*io^2;
   CPloss_diode = 0;
   SPloss_SiC = fs*(Eon_SiC+Eoff_SiC);
   SPloss_diode = fs*(Eon_diode+Eoff_diode);
else
   CPloss_SiC = 2*rdson*io*io*(1/8+m*costheta/3/pi);
   CPloss_diode = sqrt(2)*ud_plateau*io*(1/2/pi-m*costheta/8)+2*rd*io*io*(1/8-m*costheta/3/pi);
   SPloss_SiC = fs*(Eon_SiC+Eoff_SiC);
   SPloss_diode = fs*(Eon_diode+Eoff_diode);
end

CPloss_SiC = CPloss_SiC*parallel;
SPloss_SiC = SPloss_SiC*parallel;
CPloss_diode = CPloss_diode*parallel;
SPloss_diode = SPloss_diode*parallel;

if io == 0
   SPloss_SiC = 0;
   SPloss_diode = 0;
end
end

== matlab function BEV_maxSpeed/Variant Subsystem Gearbox/Gearbox Analytic/Oil Temp/MATLAB Function ==
  data: t input; P_V input; T output
function T = fcn(t, P_V)

coder.extrinsic('evalin');

% Calculate lubricant temperature
ambient_temp = 0;
ambient_temp = evalin('base', 'config_vehicle.ambient_temp');
% 
% if t < (ambient_temp - 273)
%     T = (ambient_temp - 273);
% elseif t <= 70 %Aufwärmphase mit Umgebung < t < 70°C
%     T = abs(P) * 0.0003 + rpm * 0.00004 + t; %Leistungsabhängiger und drehzahlabhängiger Energieeintrag (Temperaturanstieg)
% else %Temperatur t > 70°C -> Wärmeabgabe ~ delta_t und ~ delta_t^2 (mit delta_t = t_gearbox - t_ambient)
%     T = abs(P) * 0.0003 + rpm * 0.00004 + t - (t - ambient_temp + 273) * 0.0002 - (t - ambient_temp + 273)^2 * 0.0000022;
% end

if t < (ambient_temp - 273)
    T = (ambient_temp - 273);
elseif t <= 80 %Aufwärmphase mit Umgebung < t < 70°C
    T =0.000055*P_V + t - (t - ambient_temp + 273) * 0.0003; %Leistungsabhängiger und drehzahlabhängiger Energieeintrag (Temperaturanstieg)
else %Temperatur t > 70°C -> Wärmeabgabe ~ delta_t und ~ delta_t^2 (mit delta_t = t_gearbox - t_ambient)
    T = 0.000088*P_V + t - (t - ambient_temp + 273) * 0.0010 - (t - ambient_temp + 273)^2 * 0.000012;
end

end

== matlab function BEV_maxSpeed/Variant Subsystem Inverter/Inverter Analytic/Variant Subsystem/IM_Inverter_SiC-MOSFET_Analytic/MATLAB Function3 ==
  data: u output; T_m input; i output; usq input; usd input; costheta output; n input
function [u, i, costheta] = fcn(T_m, usq, usd, n)

   Lm = 4.5e-4;
   Lr =  0.01571 + Lm;
   p = 3;
   T_e = T_m/p;
   
   if T_m >=0
       id = -sqrt((2*T_e/p*Lr)/(3*p*Lm^2));
   else
       id = sqrt((-2*T_e/p*Lr)/(3*p*Lm^2));
   end
   iq = id;
   i = sqrt(id^2 + iq^2)/2;
   u = sqrt(usq*usq+usd*usd);
   costheta = (usd*id+usq*iq)/u/i;

   if isnan(costheta)
       costheta = 1;
   end

   if n < 0.1
       u = 0;
       i = 0;
       costheta = 1;
   end

end

== matlab function BEV_maxSpeed/Variant Subsystem Inverter/Inverter Simple/MATLAB Function ==
  data: P_inv_loss output; I_dc output; T input; n input; udc input; P_inv_total output; P_mot_total output; P_Terminal input
function [P_inv_loss, I_dc, P_inv_total, P_mot_total]= fcn(T, n, udc, P_Terminal)

    correction_faktor = 1;

    P_inv_total = P_Terminal;
    I_dc = P_inv_total/udc;
    P_mot_total = (2*T*pi*n/60+P_inv_total)/2;
    P_inv_loss = correction_faktor * (P_inv_total - P_mot_total);

end

== matlab function BEV_maxSpeed/Variant Subsystem Gearbox/Gearbox Lookup-Table/Oil Temp Gao/MATLAB Function ==
  data: t input; P input; T output; rpm input
function T = fcn(t, P, rpm)

coder.extrinsic('evalin');

% Calculate lubricant temperature
ambient_temp = 0;
ambient_temp = evalin('base', 'config_vehicle.ambient_temp');

% if t < (ambient_temp - 273)
%     T = (ambient_temp - 273);
% elseif t <= 75
%     T = abs(P) * 0.005 + t - (t - ambient_temp + 273)* 0.001;
% else
%     T = abs(P) * 0.005 + t - (t - 75) * 0.002 - (t - ambient_temp + 273)* 0.001;
% end

if t < (ambient_temp - 273)
    T = (ambient_temp - 273);
elseif t <= 70 %Aufwärmphase mit Umgebung < t < 70°C
    T = abs(P) * 0.0003 + rpm * 0.00004 + t; %Leistungsabhängiger und drehzahlabhängiger Energieeintrag (Temperaturanstieg)
else %Temperatur t > 70°C -> Wärmeabgabe ~ delta_t und ~ delta_t^2 (mit delta_t = t_gearbox - t_ambient)
    T = abs(P) * 0.0003 + rpm * 0.00004 + t - (t - ambient_temp + 273) * 0.0002 - (t - ambient_temp + 273)^2 * 0.0000022;
end

end

== matlab function BEV_maxSpeed/Variant Subsystem Gearbox/Gearbox Analytic/Variant Subsystem Analytic GB/Zweistufig_Koaxial/MATLAB Function ==
  data: P_V output double size=1; Mrad input; nrad input; Temp input; GB parameter
function P_V = Getriebe_Einstufig_Achsparallel(Mrad, nrad, Temp, GB)

if nrad == 0
    P_V = 0;
else
    P_V = Getrieberechnung_koaxial(GB,Mrad,nrad,Temp);
end

end

== matlab function BEV_maxSpeed/Variant Subsystem Inverter/Inverter Analytic/Variant Subsystem/IM_Inverter_IGBT_Analytic/MATLAB Function ==
  data: t input; udc input; w_mech input; u_sq output; u_sd output
function [u_sq, u_sd] = fcn(t, udc, w_mech)
    
    p = 3; %pole pairs
    
    V_line = udc/2;
    V_phase = V_line/sqrt(3);
    w_elect = p * w_mech;
    
    V_a = V_phase * sin(w_elect * t);
    V_b = V_phase * sin(w_elect * t - 2*pi/3);
    V_c = V_phase * sin(w_elect * t + 2*pi/3);

    % Transformation from abc to dq reference frame
    % Assuming stator flux-oriented control with d-axis aligned with rotor flux
    theta_e = w_elect * t; % Electrical angle
    
    % Clarke transformation to alpha-beta reference frame
    V_alpha = (2/3) * (V_a - 0.5 * (V_b + V_c));
    V_beta = (2/3) * ((sqrt(3)/2) * (V_b - V_c));
    
    % Park transformation to d-q reference frame
    u_sd = V_alpha * cos(theta_e) + V_beta * sin(theta_e);
    u_sq = -V_alpha * sin(theta_e) + V_beta * cos(theta_e);

end

== matlab function BEV_maxSpeed/Variant Subsystem Gearbox/Gearbox Analytic/Oil Temp Gao/MATLAB Function ==
  data: t input; P input; T output; rpm input
function T = fcn(t, P, rpm)

coder.extrinsic('evalin');

% Calculate lubricant temperature
ambient_temp = 0;
ambient_temp = evalin('base', 'config_vehicle.ambient_temp');

% if t < (ambient_temp - 273)
%     T = (ambient_temp - 273);
% elseif t <= 75
%     T = abs(P) * 0.005 + t - (t - ambient_temp + 273)* 0.001;
% else
%     T = abs(P) * 0.005 + t - (t - 75) * 0.002 - (t - ambient_temp + 273)* 0.001;
% end

if t < (ambient_temp - 273)
    T = (ambient_temp - 273);
elseif t <= 70 %Aufwärmphase mit Umgebung < t < 70°C
    T = abs(P) * 0.0003 + rpm * 0.00004 + t; %Leistungsabhängiger und drehzahlabhängiger Energieeintrag (Temperaturanstieg)
else %Temperatur t > 70°C -> Wärmeabgabe ~ delta_t und ~ delta_t^2 (mit delta_t = t_gearbox - t_ambient)
    T = abs(P) * 0.0003 + rpm * 0.00004 + t - (t - ambient_temp + 273) * 0.0002 - (t - ambient_temp + 273)^2 * 0.0000022;
end

end

== matlab function BEV_maxSpeed/Variant Subsystem Gearbox/Gearbox Analytic/Variant Subsystem Analytic GB/Zweistufig_Achsparallel/MATLAB Function ==
  data: P_V output double size=1; Mrad input; nrad input; Temp input; GB parameter
function P_V  = Getriebe_Zweistufig_Achsparallel(Mrad, nrad, Temp, GB)

if nrad == 0
    P_V = 0;
else
    [P_V] = Getrieberechnung(GB,Mrad,nrad,Temp);
end

end

== matlab function BEV_maxSpeed/Variant Subsystem Inverter/Inverter Analytic/Variant Subsystem/PMSM_Inverter_IBGT_Analytic/Analytic1 ==
  data: id_ref input; u output; i output; iq_ref input; costheta output; n input
function [u, i, costheta] =  u(id_ref,iq_ref, n)

    % Updated Motor Parameters based on provided values
    p = 6; % Number of pole pairs (from the provided data)
    psi_pm = 0.0347; % Permanent magnet flux linkage in Wb
    Ld = 0.0000436; % d-axis inductance in H
    Lq = 0.0000975; % q-axis inductance in H
    Rs = 0.0049; % Stator resistance in Ohms
    we = n*p/60*2*pi;

    is_ref = sqrt(id_ref^2 + iq_ref^2);

    isd = 1/(4*(Lq - Ld)) * (psi_pm - sqrt(psi_pm^2 + 8*is_ref^2*(Lq - Ld)^2));
    isq = sqrt(is_ref^2 - isd^2);

    usd = Rs*isd - we*Lq*isq;
    usq = Rs*isq + we*Ld*isd + we*psi_pm;
    % if u > urate*sqrt(2)
    %     if abs(n*T*2*pi/60) >= Prate
    %         Tout = Prate/(n/60*2*pi);
    %     else
    %         Tout = T;
    %     end
    %     isd = id_ref;
    %     isq = iq_ref;
    %     usd = ud_ref;
    %     usq = uq_ref;
    % end

    i = sqrt(isq*isq+isd*isd);
    u = sqrt(usq*usq+usd*usd);
    costheta = (usd*isd+usq*isq)/u/i;

    if isnan(costheta)
        costheta = 1;
    end
    if n < 0.1
        u = 0;
        i = 0;
        % Tout = 0;
        costheta = 1;
    end
    % if Tout ~= T
    %     Tout = T;
    % end
end

== matlab function BEV_maxSpeed/Variant Subsystem Inverter/Inverter Analytic/Variant Subsystem/PMSM_Inverter_SiC-MOSFET_Analytic/C2M0025120D ==
  data: io input; udc input; up input; fs input; CPloss_SiC output; CPloss_diode output; costheta input; SPloss_SiC output; SPloss_diode output; T_mosfet input; T_diode input
function [CPloss_SiC,CPloss_diode,SPloss_SiC,SPloss_diode] = SiC_MOSFET(io,udc,up,fs,costheta,T_mosfet,T_diode)
%%%%%%%%%%%%%%%%%%%%%%%%%%% parameter table %%%%%%%%%%%%%%%%%%%%%%%%%%%%%%%
%%%%%%%%%%%%%%%%%%%%%%%%%%% varialbe table %%%%%%%%%%%%%%%%%%%%%%%%%%%%%%%%
%variavle name      meaning,                                                        unit
%io,                operation current                                               (A)
%up,                operation voltage                                               (V)
%udc,               DC bus voltage,                                                 (V)
%fs,                switching frequency,                                            (Hz)
%costheta,          power factor,                                                   (none)
%CPloss_igbt,       conduction loss on IGBT,                                        (W)
%CPloss_diode,      conduction loss on the reverse paralleled diode,                (W)
%SPloss_igbt,       switching loss on IGBT,                                         (W)
%SPloss_diode,      switching loss on the reverse paralleled diode,                 (W)
%%%%%%%%%%%%%%%%%%%%%%%%%%%%%%%%%%%%%%%%%%%%%%%%%%%%%%%%%%%%%%%%%%%%%%%%%%%
parallel = 4;

io = io/parallel;
rdson_max = 0.02;       
alpha = (1.45 - 1)/(150 - 25);
ud_plateau25 = 1;                              % Fig.11; Vth,25 = 2.7
ud_plateau150 = 0.717;                         % Fig.11; Vth,150 = 2.3
%%%%%%%%%%%%%%%%%%%%%%%%%%%% linearization %%%%%%%%%%%%%%%%%%%%%%%%%%%%%%%%
rdson = rdson_max*(1 + alpha/100)^(T_mosfet - 25);
ud_plateau = ud_plateau25 + (ud_plateau25-ud_plateau150)/(25-150)*(T_diode-25);

rd = (-6 - (-3.75))/(-200 - 0) * 1.2;          % engineering calculation use safty margin value, linearization from Fig.10, using Vsd,typ = 3.5;

Eon_SiC = (0.00069/80*(io*(2/pi)))/520*udc;    % linearization from Fig.23; V_DD = 600; Eon(60, 0.0015);
Eoff_SiC = (0.001125/80*(io*(2/pi)))/520*udc;  % linearization from Fig.23; V_DD = 600; Eoff(60, 0.00075);
Eon_diode = 0;
Eoff_diode = 0;
%%%%%%%%%%%%%%%%%%%%%%%%%%%%%%%%%%%%%%%%%%%%%%%%%%%%%%%%%%%%%%%%%%%%%%%%%%%
m = sqrt(2)*up*2/udc;

if io*rdson <= ud_plateau
   CPloss_SiC = rdson*io^2;
   CPloss_diode = 0;
   SPloss_SiC = fs*(Eon_SiC+Eoff_SiC);
   SPloss_diode = fs*(Eon_diode+Eoff_diode);
else
   CPloss_SiC = 2*rdson*io*io*(1/8+m*costheta/3/pi);
   CPloss_diode = sqrt(2)*ud_plateau*io*(1/2/pi-m*costheta/8)+2*rd*io*io*(1/8-m*costheta/3/pi);
   SPloss_SiC = fs*(Eon_SiC+Eoff_SiC);
   SPloss_diode = fs*(Eon_diode+Eoff_diode);
end

CPloss_SiC = CPloss_SiC*parallel;
SPloss_SiC = SPloss_SiC*parallel;
CPloss_diode = CPloss_diode*parallel;
SPloss_diode = SPloss_diode*parallel;

if io == 0
   SPloss_SiC = 0;
   SPloss_diode = 0;
end
end

== matlab function BEV_maxSpeed/Variant Subsystem Inverter/Inverter Analytic/Variant Subsystem/PMSM_Inverter_IBGT_Analytic/Change parameters from datasheet here1 ==
  data: ic input; udc input; up input; fs input; CPloss_igbt output; CPloss_diode output; costheta input; Eon_igbt_nom input; Eoff_igbt_nom input; Erec_diode_nom input; SPloss_igbt output; SPloss_diode output; T_igbt input; T_diode input
function [CPloss_igbt,CPloss_diode,SPloss_igbt,SPloss_diode] = IGBT(ic,udc,up,fs,costheta,Eon_igbt_nom, Eoff_igbt_nom, Erec_diode_nom, T_igbt, T_diode)
%%%%%%%%%%%%%%%%%%%%%%%%%%% parameter table %%%%%%%%%%%%%%%%%%%%%%%%%%%%%%%
%%%%%%%%%%%%%%%%%%%%%%%%%%% varialbe table %%%%%%%%%%%%%%%%%%%%%%%%%%%%%%%%
% variavle name      meaning,                                                        unit
% ic,                operation current peak                                          (A)
% up,                operation voltage peak                                          (V)
% udc,               DC bus voltage,                                                 (V)
% fs,                switching frequency,                                            (Hz)
% costheta,          power factor,                                                   (none)
% CPloss_igbt,       conduction loss on IGBT,                                        (W)
% CPloss_diode,      conduction loss on the reverse paralleled diode,                (W)
% SPloss_igbt,       switching loss on IGBT,                                         (W)
% SPloss_diode,      switching loss on the reverse paralleled diode,                 (W)
%%%%%%%%%%%%%%%%%%%%%%%%%%%%%%%%%%%%%%%%%%%%%%%%%%%%%%%%%%%%%%%%%%%%%%%%%%%
parallel = 1;

ic = ic/parallel;

icn = 450;
uce_test = 400;
ifn = 450;
uf_test = 400;

T25 = 25;
T175 = 175;
uce0 = 0.75;
rc25 = 0.0005;
rc175 = 0.00089;
kCE = (rc175-rc25)/(T175-T25);
ud0 = 0.95;
rd25 = 0.00067;
rd175 = 0.00075;
kD = (rd175-rd25)/(T175-T25);
%%
rc = rc25 + (T_igbt - 25)*kCE;  
rd = rd25 + (T_diode - 25)*kD; 
uce = uce0 + ic*rc;             
uf = ud0 + ic*rd;            

m = up*sqrt(2)*2/udc; 

Eon_igbt = Eon_igbt_nom * ic/icn * udc/uce_test;    
Eoff_igbt = Eoff_igbt_nom * ic/ifn * udc/uce_test;         
Erec_diode = Erec_diode_nom * ic/ifn * udc/uf_test; 

CPloss_igbt = sqrt(2)*uce*ic*(1/2/pi+m*costheta/8) + 2*rc*ic*ic*(1/8+m*costheta/3/pi);
CPloss_diode = sqrt(2)*uf*ic*(1/2/pi-m*costheta/8) + 2*rd*ic*ic*(1/8-m*costheta/3/pi);
SPloss_igbt = fs*(Eon_igbt+Eoff_igbt);
SPloss_diode = fs*Erec_diode;

CPloss_igbt = CPloss_igbt*parallel;
CPloss_diode = CPloss_diode*parallel;
SPloss_igbt = SPloss_igbt*parallel;
SPloss_diode = SPloss_diode*parallel;

if ic == 0
    SPloss_igbt = 0;
    SPloss_diode = 0;
end
end

== matlab function BEV_maxSpeed/Variant Subsystem Inverter/Inverter Analytic/Variant Subsystem/PMSM_Inverter_SiC-MOSFET_Analytic/Analytic1 ==
  data: id_ref input; u output; i output; iq_ref input; costheta output; n input
function [u, i, costheta] =  u(id_ref,iq_ref, n)

    % Updated Motor Parameters based on provided values
    p = 6; % Number of pole pairs (from the provided data)
    psi_pm = 0.0347; % Permanent magnet flux linkage in Wb
    Ld = 0.0000436; % d-axis inductance in H
    Lq = 0.0000975; % q-axis inductance in H
    Rs = 0.0049; % Stator resistance in Ohms
    we = n*p/60*2*pi;
    urate = 142.56;

    is_ref = sqrt(id_ref^2 + iq_ref^2);

    isd = 1/(4*(Lq - Ld)) * (psi_pm - sqrt(psi_pm^2 + 8*is_ref^2*(Lq - Ld)^2));
    isq = sqrt(is_ref^2 - isd^2);

    usd = Rs*isd - we*Lq*isq;
    usq = Rs*isq + we*Ld*isd + we*psi_pm;

    i = sqrt(isq*isq+isd*isd);
    u = sqrt(usq*usq+usd*usd);
    
    if u > urate*sqrt(2)
        % if abs(n*T*2*pi/60) >= Prate
        %     Tout = Prate/(n/60*2*pi);
        % else
        %     Tout = T;
        % end
        isd = id_ref;
        isq = iq_ref;
        % usd = ud_ref;
        % usq = uq_ref;
    end

    i = sqrt(isq*isq+isd*isd);
    u = sqrt(usq*usq+usd*usd);
    costheta = (usd*isd+usq*isq)/u/i;

    if isnan(costheta)
        costheta = 1;
    end
    if n < 0.1
        u = 0;
        i = 0;
        % Tout = 0;
        costheta = 1;
    end
    % if Tout ~= T
    %     Tout = T;
    % end
end

== matlab function BEV_maxSpeed/Variant Subsystem Gearbox/Gearbox Analytic/Variant Subsystem Analytic GB/Einstufig_Achsparallel/MATLAB Function ==
  data: GB parameter; P_V output double size=1; Mrad input; nrad input; Temp input
function P_V = Getriebe_Einstufig_Achsparallel(GB, Mrad, nrad, Temp)

if nrad == 0
    P_V = 0;
else
    P_V = Getrieberechnung_Einstufig(GB,Mrad,nrad, Temp);
end

end

== matlab function BEV_maxSpeed/Variant Subsystem Inverter/Inverter Analytic/Variant Subsystem/IM_Inverter_IGBT_Analytic/Change parameters from datasheet here ==
  data: ic input; udc input; up input; fs input; CPloss_igbt output; CPloss_diode output; costheta input; Eon_igbt_nom input; Eoff_igbt_nom input; Erec_diode_nom input; SPloss_igbt output; SPloss_diode output; T_igbt input; T_diode input
function [CPloss_igbt,CPloss_diode,SPloss_igbt,SPloss_diode] = IGBT(ic,udc,up,fs,costheta,Eon_igbt_nom, Eoff_igbt_nom, Erec_diode_nom, T_igbt, T_diode)
%%%%%%%%%%%%%%%%%%%%%%%%%%% parameter table %%%%%%%%%%%%%%%%%%%%%%%%%%%%%%%
%%%%%%%%%%%%%%%%%%%%%%%%%%% varialbe table %%%%%%%%%%%%%%%%%%%%%%%%%%%%%%%%
% variavle name      meaning,                                                        unit
% ic,                operation current peak                                          (A)
% up,                operation voltage peak                                          (V)
% udc,               DC bus voltage,                                                 (V)
% fs,                switching frequency,                                            (Hz)
% costheta,          power factor,                                                   (none)
% CPloss_igbt,       conduction loss on IGBT,                                        (W)
% CPloss_diode,      conduction loss on the reverse paralleled diode,                (W)
% SPloss_igbt,       switching loss on IGBT,                                         (W)
% SPloss_diode,      switching loss on the reverse paralleled diode,                 (W)
%%%%%%%%%%%%%%%%%%%%%%%%%%%%%%%%%%%%%%%%%%%%%%%%%%%%%%%%%%%%%%%%%%%%%%%%%%%
parallel = 1;

ic = ic/parallel;

icn = 450;
uce_test = 400;
ifn = 450;
uf_test = 400;

T25 = 25;
T175 = 175;
uce0 = 0.75;
rc25 = 0.0005;
rc175 = 0.00089;
kCE = (rc175-rc25)/(T175-T25);
ud0 = 0.95;
rd25 = 0.00067;
rd175 = 0.00075;
kD = (rd175-rd25)/(T175-T25);
%%
rc = rc25 + (T_igbt - 25)*kCE;  
rd = rd25 + (T_diode - 25)*kD; 
uce = uce0 + ic*rc;             
uf = ud0 + ic*rd;            

m = up*sqrt(2)*2/udc; 

Eon_igbt = Eon_igbt_nom * ic/icn * udc/uce_test;    
Eoff_igbt = Eoff_igbt_nom * ic/ifn * udc/uce_test;         
Erec_diode = Erec_diode_nom * ic/ifn * udc/uf_test; 

CPloss_igbt = sqrt(2)*uce*ic*(1/2/pi+m*costheta/8) + 2*rc*ic*ic*(1/8+m*costheta/3/pi);
CPloss_diode = sqrt(2)*uf*ic*(1/2/pi-m*costheta/8) + 2*rd*ic*ic*(1/8-m*costheta/3/pi);
SPloss_igbt = fs*(Eon_igbt+Eoff_igbt);
SPloss_diode = fs*Erec_diode;

CPloss_igbt = CPloss_igbt*parallel;
CPloss_diode = CPloss_diode*parallel;
SPloss_igbt = SPloss_igbt*parallel;
SPloss_diode = SPloss_diode*parallel;

if ic == 0
    SPloss_igbt = 0;
    SPloss_diode = 0;
end
end
